simulink model "test_sim"  (R2018b)
settings: Solver=VariableStepAuto  StartTime=0.0  StopTime=10.0  RelTol=1e-3
values from neighbouring files (symbols this model uses):
  KLQG1 = lqg(sys,QXU,QWV,QI,'1dof')    [test.m]
  sys = tf(num,den)    [bod_plot.m]    (also in nyq_plot.m; test.m = ss(A,B,C,D))
settings Model: Creator=eshojaei  LastModifiedBy=eshojaei

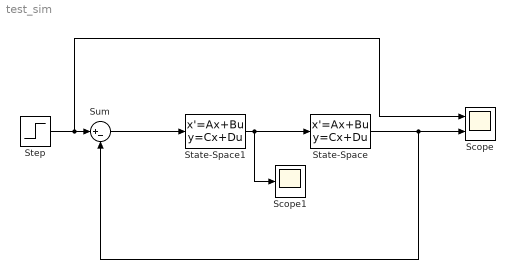
== system test_sim ==
  Scope : Scope  NumInputPorts=2
  Scope1 : Scope
  State-Space : StateSpace  A=sys.A  B=sys.B  C=sys.C  D=sys.D  InitialCondition=0
  State-Space1 : StateSpace  A=KLQG1.A  B=KLQG1.B  C=KLQG1.C  D=KLQG1.D  InitialCondition=0
  Step : Step  SampleTime=0
  Sum : Sum  Inputs=|+-
  wires:
  State-Space/1 -> Scope/2, Sum/2
  Sum/1 -> State-Space1/1
  State-Space1/1 -> Scope1/1, State-Space/1
  Step/1 -> Scope/1, Sum/1
